simulink model "Model_Sim"  (R2024b)
settings: Solver=ode4  StartTime=0.0  StopTime=20  FixedStep=0.01  RelTol=1e-3
values from neighbouring files (symbols this model uses):
  hat_A = diag(best_pop(1:3))    [Model_identification.m]
  hat_B = diag(best_pop(4:6))    [Model_identification.m]
settings Model: Creator=wook9  LastModifiedBy=junso
settings RTWCC: GPUComputeCapability=3.5

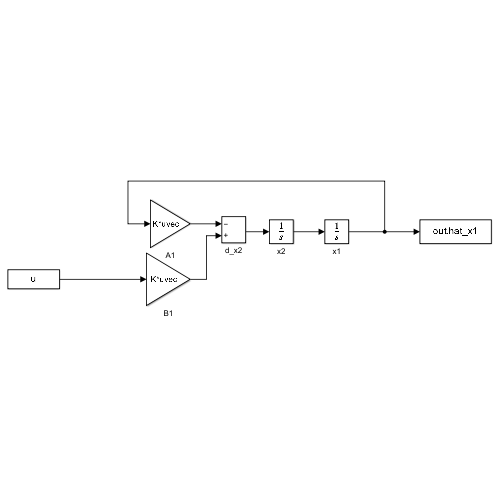
[thumbnail: Simulink's stored preview of the top-level diagram]
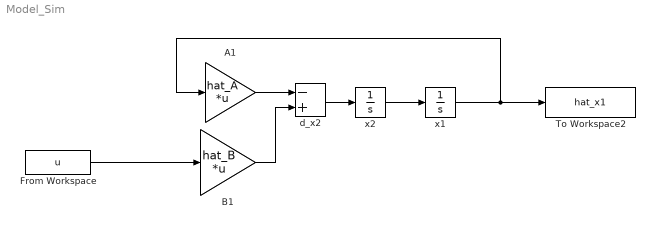
== system Model_Sim ==
  A1 : Gain  Gain=hat_A  Multiplication=Matrix(K*u) (u vector)
  B1 : Gain  Gain=hat_B  Multiplication=Matrix(K*u) (u vector)
  From Workspace : FromWorkspace  VariableName=u
  To Workspace2 : ToWorkspace  VariableName=hat_x1  SampleTime=-1
      settings: Save2DSignal=2-D array (concatenate along first dimension)
  d_x2 : Sum  Inputs=-+
  x1 : Integrator
  x2 : Integrator
  wires:
  x1/1 -> A1/1, To Workspace2/1
  x2/1 -> x1/1
  d_x2/1 -> x2/1
  A1/1 -> d_x2/1
  From Workspace/1 -> B1/1
  B1/1 -> d_x2/2
